simulink model "rtwdemo_dynamicio"  (Simulink 6.0)
settings: Solver=FixedStepDiscrete  StartTime=0.0  StopTime=1  FixedStep=1  RelTol=1e-3
PostLoadFcn:
  | clear;K=Simulink.Parameter;K.Value=2;K.RTWInfo.StorageClass='SimulinkGlobal';
libraries: rtwdemowidgets x2
settings Model: Creator=The MathWorks Inc.  LastModifiedBy=batserve  ExtModeAutoUpdateStatusClock=off  ProdHWDeviceType=32-bit Embedded Processor
settings DataIOCC: LimitDataPoints=off  SaveOutput=off  SaveTime=off  SignalLoggingName=logsOut
settings OptimizationCC: InlineParams=on  EnforceIntegerDowncast=off  StateBitsets=on  DataBitsets=on  UseTempVars=on
settings DebuggingCC: CheckExecutionContextPreStartOutputMsg=on  CheckExecutionContextRuntimeOutputMsg=on  SolverPrmCheckMsg=none
settings HardwareCC: ProdHWDeviceType=32-bit Embedded Processor  TargetHWDeviceType=32-bit Generic  ProdEqTarget=off
settings ModelReferenceCC: UpdateModelReferenceTargets=IfOutOfDate
settings RTWCC: Description=RTW Embedded Coder (no auto configuration)  GenerateReport=on  RTWVerbose=off  ProcessScript=grt_make_rtw_hook  LaunchReport=on
settings CodeAppCC: ForceParamTrailComments=on
settings GRTTargetCC: MatFileLogging=off

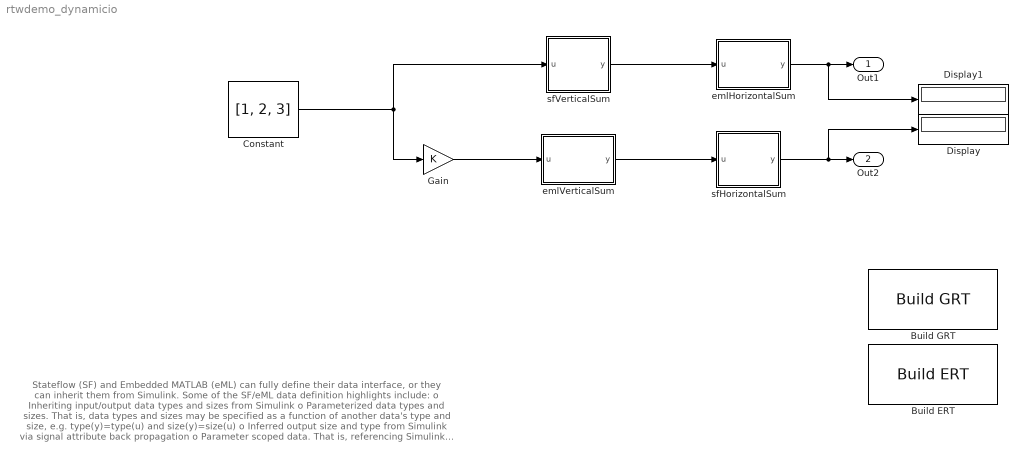
== system rtwdemo_dynamicio ==
  note: Stateflow (SF) and Embedded MATLAB (eML) can fully define their data interface, or they can
      | inherit them from Simulink.  Some of the SF/eML data definition highlights include:
      |
      | o Inheriting input/output data types and sizes from Simulink
      | o Parameterized data types and sizes.  That is, data types and sizes may be specified
      |   as a function of another data's type and size, e.g. type(y)=type(u) and size(y)=size(u)
      | o Inferred output size and type from Simulink via signal attribute back propagation
      | o Parameter scoped data.  That is, referencing Simulink parameters in SF and eML
      |
      | In this example:
      |
      | o The data type and size of all SF/eML data is inherited from Simulink
      | o The Gain block and SF chart sfVerticalSum share the Simulink parameter K, which is
      |    defined in the MATLAB Workspace as a Simulink.Parameter with SimulinkGlobal storage
      |    class (i.e., rtP.K in the generated code)
      |
      | Some exercises to try:
      |
      | o Compile the model (Edit->Update Diagram) and note the displayed signal types and sizes
      | o Change the data type and/or size of the Constant block and recompile the model.  Note
      |    the attributes of the signals automatically adapt to the constant block specification
      | o Generate and inspect code using the blue buttons to the right.  Note that K is shared
      |    by the Gain and sfVerticalSum block.
  Build ERT : rtwdemowidgets/Build ERT  attrib_overrides={}
  Build GRT : rtwdemowidgets/Build GRT  attrib_overrides={}
  Constant : Constant  Value=[1, 2, 3]  VectorParams1D=off  OutDataTypeMode=single
  Display : Display
  Display1 : Display
  Gain : Gain  Gain=K
  emlHorizontalSum : Stateflow chart  PropExecContextAcrossSSBoundary=on
  emlVerticalSum : Stateflow chart  PropExecContextAcrossSSBoundary=on
  sfHorizontalSum : Stateflow chart  PropExecContextAcrossSSBoundary=on
  sfVerticalSum : Stateflow chart  PropExecContextAcrossSSBoundary=on
  Out1 : Outport
  Out2 : Outport  Port=2
  wires:
  emlVerticalSum/1(y) -> sfHorizontalSum/1(u)
  sfHorizontalSum/1(y) -> Out2/1, Display/1
  sfVerticalSum/1(y) -> emlHorizontalSum/1(u)
  emlHorizontalSum/1(y) -> Out1/1, Display1/1
  Gain/1 -> emlVerticalSum/1(u)
  Constant/1 -> sfVerticalSum/1(u), Gain/1

== matlab function emlHorizontalSum ==
  data: u input inherited; y output type(u)
function y = fcn(u)
y = sum(u,2);

== matlab function emlVerticalSum ==
  data: u input inherited; y output type(u)
function y = fcn(u)
y = sum(u,1);

== matlab function sfHorizontalSum ==
  data: u1 function_input type(u) size=size(u); y1 function_output type(u) size=[size(u,1) 1]; u input inherited; y output type(u) size=[size(u,1),1]
function y1 = f(u1)
y1 = sum(u1,2);

== matlab function sfVerticalSum ==
  data: u1 function_input type(u) size=size(u); y1 function_output type(u) size=[1 size(u,2)]; u input inherited; y output type(u) size=[1,size(u,2)]; K parameter type(u)
function y1 = f(u1)
y1 = sum(u1,1);
